simulink model "Q3b_12_pulse_rectifier"  (R2018a)
settings: Solver=VariableStepDiscrete  StartTime=0.0  StopTime=1  RelTol=1e-3
undefined symbols (not defined in the file): D11, Delta
libraries: powerlib x11, dspstat3 x2, powerlib_meascontrol x1
settings Model: Creator=bulbu  LastModifiedBy=bulbu

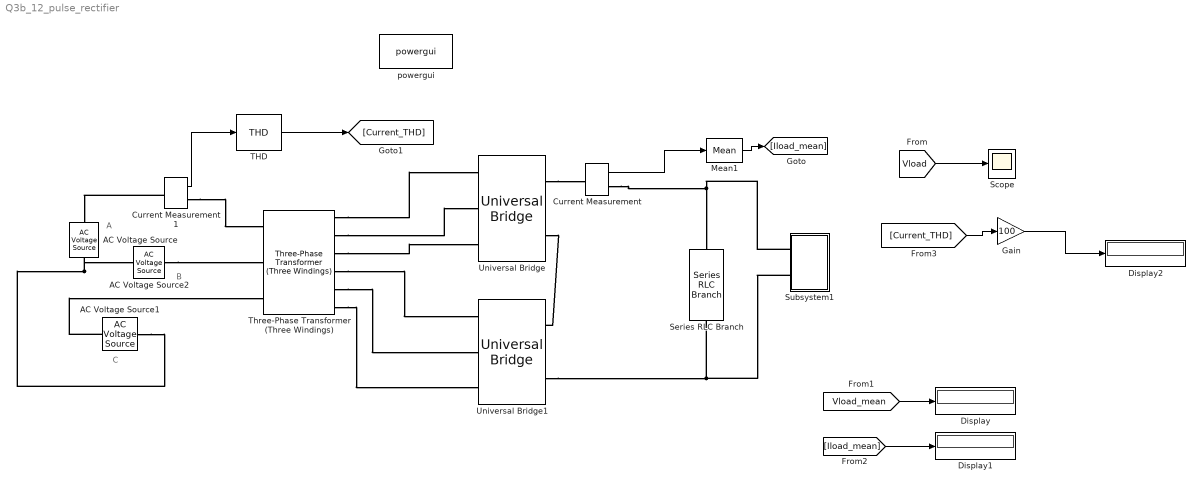
== system Q3b_12_pulse_rectifier ==
  note: B
  note: A
  note: C
  AC Voltage Source : powerlib/Electrical Sources/AC Voltage Source  Amplitude=326.6  Phase=0  Frequency=50  SampleTime=0  Measurements=None  BusType=swing  Pref=10e3  Qref=0  Qmin=-inf  Qmax=+inf
  AC Voltage Source1 : powerlib/Electrical Sources/AC Voltage Source  Amplitude=326.6  Phase=-120  Frequency=50  SampleTime=0  Measurements=None  BusType=swing  Pref=10e3  Qref=0  Qmin=-inf  Qmax=+inf
  AC Voltage Source2 : powerlib/Electrical Sources/AC Voltage Source  Amplitude=326.6  Phase=120  Frequency=50  SampleTime=0  Measurements=None  BusType=swing  Pref=10e3  Qref=0  Qmin=-inf  Qmax=+inf
  Current Measurement : powerlib/Measurements/Current Measurement  PhasorSimulation=off  OutputType=Complex  PSBequivalent=0
  Current Measurement1 : powerlib/Measurements/Current Measurement  PhasorSimulation=off  OutputType=Complex  PSBequivalent=0
  Display : Display
  Display1 : Display
  Display2 : Display
  Gain : Gain  Gain=100
  Mean1 : dspstat3/Mean  run=on  InputProcessing=Columns as channels (frame based)  reset_popup=None  directionMode=Each column  dimension=1  roiEnable=off  roiType=Rectangles  roiPortion=Entire ROI  roiOutput=Individual statistics for each ROI  roiFlag=off  roundingMode=Floor  overflowMode=off  outputDataTypeStr=Inherit: Same as accumulator  outputMin=[]  outputMax=[]  outputLastDataTypeStr=Inherit: Same as accumulator
  Scope : Scope
  Series RLC Branch : powerlib/Elements/Series RLC Branch  LConnTagsString=__new0  RConnTagsString=__new0  BranchType=R  Resistance=10  Inductance=1e-3  SetiL0=off  InitialCurrent=0  Capacitance=1e-6  Setx0=off  InitialVoltage=0  Measurements=None
  Subsystem1 : Subsystem
  THD : powerlib_meascontrol/Measurements/THD  Freq=50  Ts=1e-06
  Three-Phase Transformer (Three Windings) : powerlib/Elements/Three-Phase Transformer (Three Windings)  Winding1Connection=Delta (D11)  Winding2Connection=Y  Winding3Connection=Delta (D11)  CoreType=Three single-phase transformers  SetSaturation=off  Hysteresis=off  DataFile='hysteresis'  SetInitialFlux=off  Measurements=None  UNITS=pu  NominalPower=[ 250e6 , 50 ]  Winding1=[400, 0.002 , 0.08 ]  Winding2=[200 , 0.002 , 0.08 ]  Winding3=[ 200 , 0.002 , 0.08 ]  Rm=500  Lm=500  L0=0.5  Saturation=[ 0,0 ; 0.0024,1.2 ; 1.0,1.52 ]  InitialFluxes=[0.8 -0.8 0.7]  MoreParameters=off  BreakLoop=off  DataType=off  TransfoNumber=1
      settings: SourceProductName=Simscape Power Systems  SourceProductBaseCode=PS
  Universal Bridge : powerlib/Power Electronics/Universal Bridge  Arms=3  SnubberResistance=1e5  SnubberCapacitance=inf  Device=Diodes  Ron=1e-3  Lon=0  ForwardVoltages="[  0  0  ]"  ForwardVoltage=0  GTOparameters=[ 10e-6 , 20e-6 ]  IGBTparameters=[ 1e-6 , 2e-6 ]  Measurements=None  Measurements_2=None  converterType=Rectifier
  Universal Bridge1 : powerlib/Power Electronics/Universal Bridge  Arms=3  SnubberResistance=1e5  SnubberCapacitance=inf  Device=Diodes  Ron=1e-3  Lon=0  ForwardVoltages="[  0  0  ]"  ForwardVoltage=0  GTOparameters=[ 10e-6 , 20e-6 ]  IGBTparameters=[ 1e-6 , 2e-6 ]  Measurements=None  Measurements_2=None  converterType=Rectifier
  powergui : powerlib/powergui  Priority=1  SimulationMode=Discrete  SampleTime=1e-6  frequency=60  Iterations=50  frequencyindice=50  Pbase=100e6  ErrMax=1e-4  UnitsV=kV  UnitsW=MW  buscounter=0  FunctionMessages=off  echomessages=off  EnableUseOfTLC=off  CurrentSourceSwitches=off  DisableSnubberDevices=off  DisableRonSwitches=off  DisableVfSwitches=off  DisplayEquations=off  SolverType=Tustin/Backward Euler (TBE)  Interpol=off  ExternalGateDelay=off  methode=off  Ts=100  x0status=blocks  SPID=on  SwTol=0  HookPort=off  RestoreLinks=warning  ResistiveCurrentMeasurement=off  Frange=[0:2:500]  Ylog=off  Xlog=on  ShowGrid=off  save=off  variable=ZData  structure=0  ZoomFFT=off  StartTime=0.0  cycles=1  DisplayStyle=1  fundamental=60  FreqAxis=off  MaxFrequency=1000  frequencyindicesteady=1  RmsSteady=1  display=off
  wires:
  [Vload] -> Scope/1
  [Vload_mean] -> Display/1
  Current Measurement/1 -> Mean1/1
  Mean1/1 -> [Iload_mean]
  [Iload_mean] -> Display1/1
  Current Measurement1/1 -> THD/1
  THD/1 -> [Current_THD]
  [Current_THD] -> Gain/1
  Gain/1 -> Display2/1
  connections:
  Three-Phase Transformer (Three Windings)/RConn1 -- Universal Bridge/LConn1
  Three-Phase Transformer (Three Windings)/RConn2 -- Universal Bridge/LConn2
  Three-Phase Transformer (Three Windings)/RConn3 -- Universal Bridge/LConn3
  Three-Phase Transformer (Three Windings)/RConn4 -- Universal Bridge1/LConn1
  Three-Phase Transformer (Three Windings)/RConn5 -- Universal Bridge1/LConn2
  Three-Phase Transformer (Three Windings)/RConn6 -- Universal Bridge1/LConn3
  Universal Bridge/RConn2 -- Universal Bridge1/RConn1
  Subsystem1/LConn1 -- Current Measurement/RConn1 -- Series RLC Branch/RConn1
  Universal Bridge1/RConn2 -- Subsystem1/LConn2 -- Series RLC Branch/LConn1
  AC Voltage Source1/LConn1 -- AC Voltage Source2/LConn1 -- AC Voltage Source/LConn1
  Universal Bridge/RConn1 -- Current Measurement/LConn1
  AC Voltage Source2/RConn1 -- Three-Phase Transformer (Three Windings)/LConn2
  AC Voltage Source1/RConn1 -- Three-Phase Transformer (Three Windings)/LConn3
  Current Measurement1/LConn1 -- AC Voltage Source/RConn1
  Current Measurement1/RConn1 -- Three-Phase Transformer (Three Windings)/LConn1

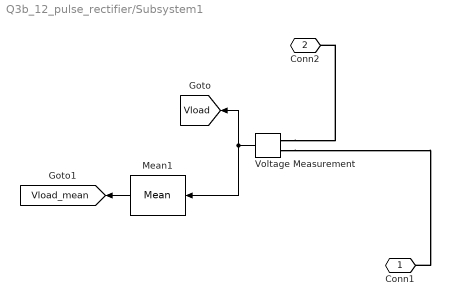
== system Q3b_12_pulse_rectifier/Subsystem1 ==
  Mean1 : dspstat3/Mean  run=on  InputProcessing=Columns as channels (frame based)  reset_popup=None  directionMode=Each column  dimension=1  roiEnable=off  roiType=Rectangles  roiPortion=Entire ROI  roiOutput=Individual statistics for each ROI  roiFlag=off  roundingMode=Floor  overflowMode=off  outputDataTypeStr=Inherit: Same as accumulator  outputMin=[]  outputMax=[]  outputLastDataTypeStr=Inherit: Same as accumulator
  Voltage Measurement : powerlib/Measurements/Voltage Measurement  PhasorSimulation=off  OutputType=Complex  PSBequivalent=0
  Conn1 : PMIOPort  Side=Left
  Conn2 : PMIOPort  Port=2  Side=Left
  tag scope: Vload=global, Vload_mean=global
  wires:
  Voltage Measurement/1 -> Mean1/1, [Vload]
  Mean1/1 -> [Vload_mean]
  connections:
  Voltage Measurement/LConn2 -- Conn2/RConn1
  Voltage Measurement/LConn1 -- Conn1/RConn1
